simulink model "SystRefAnalogique"  (Simulink 10.3)
settings: Solver=FixedStepDiscrete  StartTime=0.0  StopTime=8.75  RelTol=1e-3  EnableMultiTasking=on
libraries: dsparch4 x3, dspsigops x1, dspsrcs4 x1
settings Model: Creator=sebastienroy  LastModifiedBy=sebastienroy  MultithreadedSim=on
settings DataIOCC: LimitDataPoints=on  SignalLoggingSaveFormat=Dataset
settings OptimizationCC: ExpressionDepthLimit=128
settings DebuggingCC: SolverPrmCheckMsg=warning  FcnCallInpInsideContextMsg=error
settings GRTTargetCC: CombineOutputUpdateFcns=on  GRTInterface=off

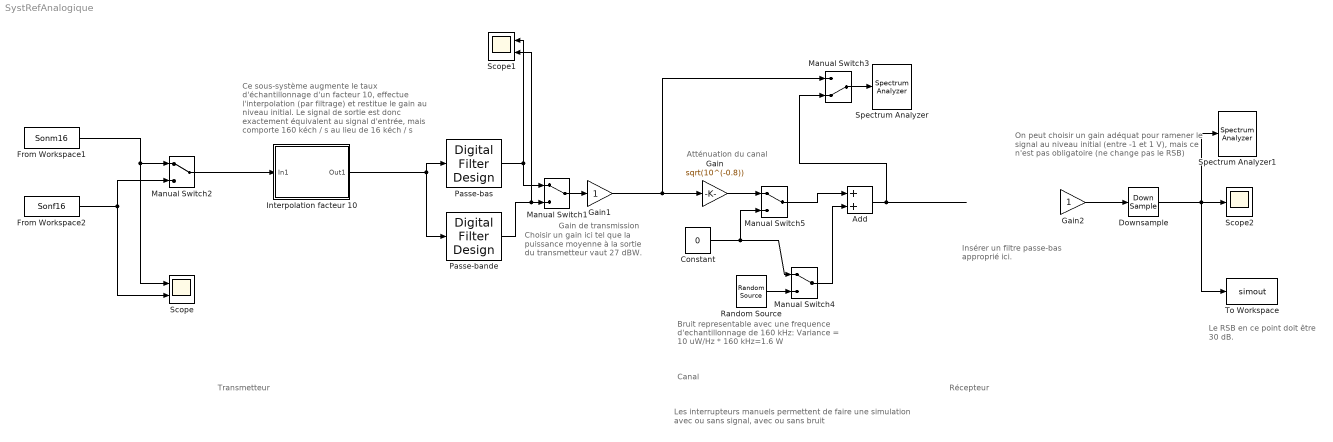
== system SystRefAnalogique ==
  note: Transmetteur
  note: Les interrupteurs manuels permettent de faire une simulation
      | avec ou sans signal, avec ou sans bruit
  note: Récepteur
  note: Canal
  note: Choisir un gain ici tel que
      | la puissance moyenne à la
      | sortie du transmetteur vaut
      | 27 dBW.
  note: Le RSB en ce point doit
      | être 30 dB.
  note: On peut choisir un gain adéquat pour ramener
      | le signal au niveau initial (entre -1 et 1 V), mais
      | ce n'est pas obligatoire (ne change pas le RSB)
  note: Insérer un filtre passe-bas
      | approprié ici.
  note: Ce sous-système augmente le taux
      | d'échantillonnage d'un facteur 10, effectue
      | l'interpolation (par filtrage) et restitue le gain
      | au niveau initial. Le signal de sortie est donc
      | exactement équivalent au signal d'entrée, mais
      | comporte 160 kéch / s au lieu de 16 kéch / s
  note: Atténuation du canal
  note: Gain de transmission
  note: Bruit representable avec une frequence
      | d'echantillonnage de 160 kHz:
      | Variance = 10 uW/Hz * 160 kHz=1.6 W
  Add : Sum
  Constant : Constant  Value=0
  Downsample : DownSample  N=10  RateOptions=Allow multirate processing
  From Workspace1 : FromWorkspace  VariableName=Sonm16  SampleTime=1/16000  Interpolate=off  OutputAfterFinalValue=Setting to zero
  From Workspace2 : FromWorkspace  VariableName=Sonf16  SampleTime=1/16000  Interpolate=off  OutputAfterFinalValue=Setting to zero
  Gain : Gain  Gain=sqrt(10^(-0.8))
  Gain1 : Gain
  Gain2 : Gain
  Interpolation facteur 10 : Subsystem
  Manual Switch{1..2,4..5} (4 alike) : ManualSwitch
  Manual Switch3 : ManualSwitch  CurrentSetting=0
  Passe-bande : dsparch4/Digital Filter Design  mwdsp_browser_bugfix_var=off
  "Passe-bas " : dsparch4/Digital Filter Design  mwdsp_browser_bugfix_var=off
  Random Source : dspsrcs4/Random Source  SrcType=Gaussian  NormMethod=Ziggurat  CltLength=12  MinVal=0  MaxVal=1  MeanVal=0  VarVal=1.6  RepMode=Not repeatable  rawSeed=1  IsInherit=on  SampMode=Discrete  SampTime=1  SampFrame=1  DataType=Double  OutComplex=Real  OutputFrames=on
  Scope : Scope  NumInputPorts=2
  Scope1 : Scope  NumInputPorts=2
  Scope2 : Scope
  Spectrum Analyzer : SpectrumAnalyzer
  Spectrum Analyzer1 : SpectrumAnalyzer
  To Workspace : ToWorkspace  VariableName=simout  SampleTime=-1
      settings: Save2DSignal=2-D array (concatenate along first dimension)
  wires:
  "Passe-bas "/1 -> Manual Switch1/1, Scope1/1
  Passe-bande/1 -> Manual Switch1/2, Scope1/2
  Manual Switch1/1 -> Gain1/1
  Add/1 -> Manual Switch3/2
  ? -> Gain2/1
  Manual Switch3/1 -> Spectrum Analyzer/1
  From Workspace1/1 -> Scope/1, Manual Switch2/1
  From Workspace2/1 -> Manual Switch2/2, Scope/2
  Downsample/1 -> To Workspace/1, Scope2/1, Spectrum Analyzer1/1
  Gain1/1 -> Gain/1, Manual Switch3/1
  Random Source/1 -> Manual Switch4/2
  Manual Switch4/1 -> Add/2
  Manual Switch5/1 -> Add/1
  Constant/1 -> Manual Switch5/2, Manual Switch4/1
  Gain2/1 -> Downsample/1
  Interpolation facteur 10/1(Out1) -> "Passe-bas "/1, Passe-bande/1
  Manual Switch2/1 -> Interpolation facteur 10/1(In1)
  Gain/1 -> Manual Switch5/1

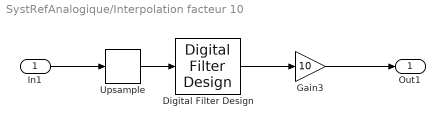
== system SystRefAnalogique/Interpolation facteur 10 ==
  In1 : Inport
  Digital Filter Design : dsparch4/Digital Filter Design  mwdsp_browser_bugfix_var=off
  Gain3 : Gain  Gain=10
  Upsample : dspsigops/Upsample  N=10  phase=0  RateOptions=Allow multirate processing  ic=0  mode=Unused parameter value
  Out1 : Outport
  wires:
  Gain3/1 -> Out1/1
  In1/1 -> Upsample/1
  Digital Filter Design/1 -> Gain3/1
  Upsample/1 -> Digital Filter Design/1
